simulink model "validazione_sonar_front"  (R2018b)
settings: Solver=VariableStepAuto  StartTime=0.0  StopTime=5.0  RelTol=1e-3
values from neighbouring files (symbols this model uses):
  p_sonar_front = [a;0;0]    [init_sensors.m]
  tilt_front = deg2rad(45)    [init_sensors.m]
  Ts_sonar_front = 0.5    [init_sensors.m]
libraries: simulink x2
settings Model: Creator=chiara-s  LastModifiedBy=chiara-s

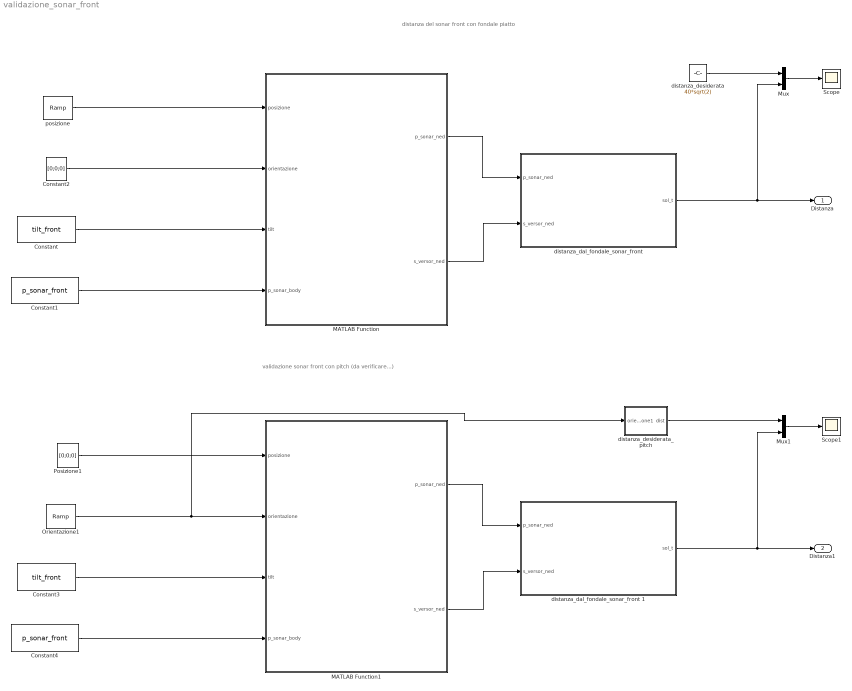
== system validazione_sonar_front ==
  note: validazione sonar front con pitch (da verificare...)
  note: distanza del sonar front con fondale piatto
  Constant : Constant  Value=tilt_front  VectorParams1D=off  SampleTime=Ts_sonar_front
  Constant1 : Constant  Value=p_sonar_front  VectorParams1D=off  SampleTime=Ts_sonar_front
  Constant2 : Constant  Value=[0;0;0]  VectorParams1D=off
  Constant3 : Constant  Value=tilt_front  VectorParams1D=off  SampleTime=Ts_sonar_front
  Constant4 : Constant  Value=p_sonar_front  VectorParams1D=off  SampleTime=Ts_sonar_front
  MATLAB Function : MATLAB Function  TreatAsAtomicUnit=on
  MATLAB Function1 : MATLAB Function  TreatAsAtomicUnit=on
  Mux : Mux  Inputs=2
  Mux1 : Mux  Inputs=2
  Orientazione1 : simulink/Sources/Ramp  slope=[0;2*pi/180;0]  start=0  InitialOutput=[0;0;0]  VectorParams1D=off
  Posizione1 : Constant  Value=[0;0;0]  VectorParams1D=off
  Scope : Scope
  Scope1 : Scope
  "distanza_dal_fondale_sonar_front " : MATLAB Function  TreatAsAtomicUnit=on
  distanza_dal_fondale_sonar_front 1 : MATLAB Function  TreatAsAtomicUnit=on
  distanza_desiderata : Constant  Value=40*sqrt(2)
  distanza_desiderata_pitch : MATLAB Function  TreatAsAtomicUnit=on
  posizione : simulink/Sources/Ramp  slope=[40;40;0]  start=0  InitialOutput=[0;0;0]  VectorParams1D=off
  Distanza : Outport
  Distanza1 : Outport  Port=2
  wires:
  Constant/1 -> MATLAB Function/3(tilt)
  Constant2/1 -> MATLAB Function/2(orientazione)
  MATLAB Function/2(s_versor_ned) -> "distanza_dal_fondale_sonar_front "/2(s_versor_ned)
  Constant1/1 -> MATLAB Function/4(p_sonar_body)
  MATLAB Function/1(p_sonar_ned) -> "distanza_dal_fondale_sonar_front "/1(p_sonar_ned)
  posizione/1 -> MATLAB Function/1(posizione)
  "distanza_dal_fondale_sonar_front "/1(sol_t) -> Mux/2, Distanza/1
  distanza_desiderata/1 -> Mux/1
  Mux/1 -> Scope/1
  Constant3/1 -> MATLAB Function1/3(tilt)
  distanza_desiderata_pitch/1(dist) -> Mux1/1
  Constant4/1 -> MATLAB Function1/4(p_sonar_body)
  MATLAB Function1/1(p_sonar_ned) -> distanza_dal_fondale_sonar_front 1/1(p_sonar_ned)
  distanza_dal_fondale_sonar_front 1/1(sol_t) -> Mux1/2, Distanza1/1
  MATLAB Function1/2(s_versor_ned) -> distanza_dal_fondale_sonar_front 1/2(s_versor_ned)
  Mux1/1 -> Scope1/1
  Posizione1/1 -> MATLAB Function1/1(posizione)
  Orientazione1/1 -> MATLAB Function1/2(orientazione), distanza_desiderata_pitch/1(orientazione1)

== matlab function validazione_sonar_front/MATLAB Function1 ==
  data: posizione input; p_sonar_ned output; orientazione input; s_versor_ned output; tilt input; p_sonar_body input
function [p_sonar_ned, s_versor_ned] = rot_body_ned(posizione,orientazione,tilt,p_sonar_body)
   
 roll = orientazione(1)
 pitch = orientazione(2)
 yaw = orientazione(3)
 xNorth = posizione(1)
 yEast = posizione(2)
 zDown = posizione(3)
 Rx = [1 0 0; 0 cos(roll) -sin(roll); 0 sin(roll) cos(roll)];
 Ry = [cos(pitch) 0 sin(pitch); 0 1 0; -sin(pitch) 0 cos(pitch)];
 Rz = [cos(yaw) -sin(yaw) 0; sin(yaw) cos(yaw) 0; 0 0 1];
 J1 = Rz*Ry*Rx; %matrice di rotazione da body a ned frame 

 s_versor_body = [sin(tilt); 0 ; cos(tilt)];	% direzione sonar in terna body
 s_versor_ned = J1*s_versor_body;
 
 cs2sensor_ned = J1*p_sonar_body; % distanza cds-sensore in Ned
 %Posizione sensore in Ned frame:
 p_sonar_ned = [xNorth; yEast; zDown] + cs2sensor_ned;
end

== matlab function validazione_sonar_front/distanza_dal_fondale_sonar_front 1 ==
  data: p_sonar_ned input; sol_t output; s_versor_ned input
function sol_t = sonar_down(p_sonar_ned, s_versor_ned)

coder.extrinsic('fondale_piatto');
sol_t = 0;
sol_t = fondale_piatto(p_sonar_ned, s_versor_ned)

end

== matlab function validazione_sonar_front/distanza_desiderata_pitch ==
  data: orientazione1 input; dist output
function dist = beccheggio(orientazione1)

h = 40 ; % distanza del sonar dal fondale

dist = 0;
dist = h/cos(orientazione1(2)+pi/4);

end

== matlab function validazione_sonar_front/MATLAB Function ==
  data: posizione input; p_sonar_ned output; orientazione input; s_versor_ned output; tilt input; p_sonar_body input
function [p_sonar_ned, s_versor_ned] = rot_body_ned(posizione,orientazione,tilt,p_sonar_body)
   
 roll = orientazione(1)
 pitch = orientazione(2)
 yaw = orientazione(3)
 xNorth = posizione(1)
 yEast = posizione(2)
 zDown = posizione(3)
 Rx = [1 0 0; 0 cos(roll) -sin(roll); 0 sin(roll) cos(roll)];
 Ry = [cos(pitch) 0 sin(pitch); 0 1 0; -sin(pitch) 0 cos(pitch)];
 Rz = [cos(yaw) -sin(yaw) 0; sin(yaw) cos(yaw) 0; 0 0 1];
 J1 = Rz*Ry*Rx; %matrice di rotazione da body a ned frame 

 s_versor_body = [sin(tilt); 0 ; cos(tilt)];	% direzione sonar in terna body
 s_versor_ned = J1*s_versor_body;
 
 cs2sensor_ned = J1*p_sonar_body; % distanza cds-sensore in Ned
 %Posizione sensore in Ned frame:
 p_sonar_ned = [xNorth; yEast; zDown] + cs2sensor_ned;
end

== matlab function validazione_sonar_front/distanza_dal_fondale_sonar_front  ==
  data: p_sonar_ned input; sol_t output; s_versor_ned input
function sol_t = sonar_down(p_sonar_ned, s_versor_ned)

coder.extrinsic('fondale_piatto');
sol_t = 0;
sol_t = fondale_piatto(p_sonar_ned, s_versor_ned)

end
